simulink model "B_durham_incremental_example"  (R2017a)
settings: Solver=FixedStepAuto  StartTime=0.0  StopTime=10.0  FixedStep=1  RelTol=1e-3
settings Model: Creator=Luca  LastModifiedBy=Luca

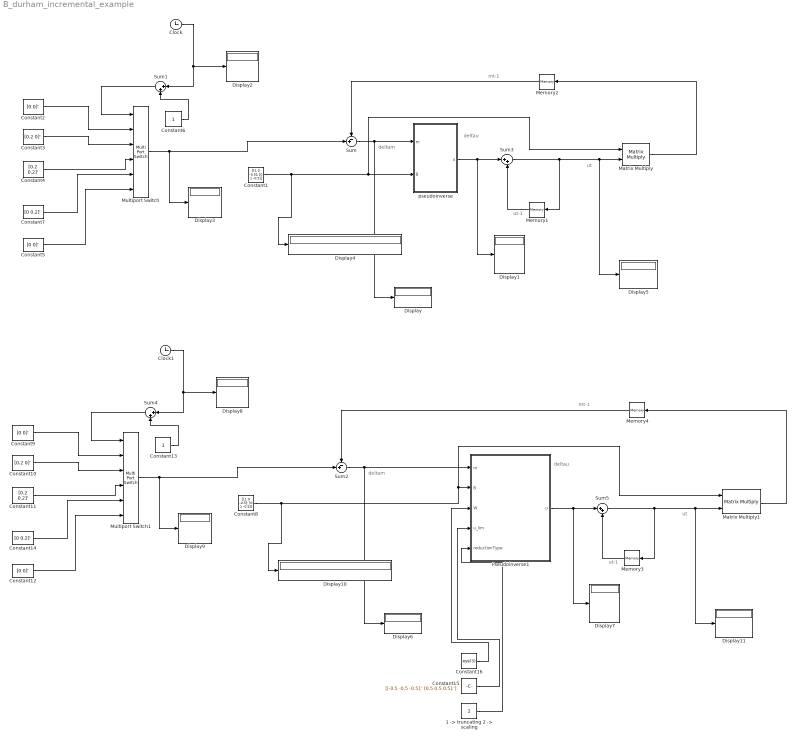
== system B_durham_incremental_example ==
  note: deltam
  note: deltau
  note: ut
  note: ut-1
  note: mt-1
  note: deltam
  note: ut
  note: ut-1
  note: deltau
  note: mt-1
  "1 -> truncating 2 -> scaling" : Constant  Value=2
  Clock : Clock
  Clock1 : Clock
  Constant1 : Constant  Value=[[1 0 -0.5]; [0 1 -0.5]]
  Constant10 : Constant  Value=[0.2 0]'
  Constant11 : Constant  Value=[0.2 0.2]'
  Constant{2,5,9,12} (4 alike) : Constant  Value=[0 0]'
  Constant13 : Constant
  Constant14 : Constant  Value=[0 0.2]'
  Constant15 : Constant  Value=[[-0.5 -0.5 -0.5].' [0.5 0.5 0.5].']
  Constant16 : Constant  Value=eye(3)
  Constant3 : Constant  Value=[0.2 0]'
  Constant4 : Constant  Value=[0.2 0.2]'
  Constant6 : Constant
  Constant7 : Constant  Value=[0 0.2]'
  Constant8 : Constant  Value=[[1 0 -0.5]; [0 1 -0.5]]
  Display{,1..11} (12 alike) : Display
  Matrix Multiply : Product  Multiplication=Matrix(*)
  Matrix Multiply1 : Product  Multiplication=Matrix(*)
  Memory{1..4} (4 alike) : Memory
  Multiport Switch : MultiPortSwitch  Inputs=5
  Multiport Switch1 : MultiPortSwitch  Inputs=5
  Pseudoinverse1 : MATLAB Function  TreatAsAtomicUnit=on
  Sum : Sum  Inputs=-+|
  Sum{1,3..5} (4 alike) : Sum  Inputs=|++
  Sum2 : Sum  Inputs=-+|
  pseudoinverse : MATLAB Function  TreatAsAtomicUnit=on
  wires:
  Memory1/1 -> Sum3/2
  Sum/1 -> Display/1, pseudoinverse/1(m)
  pseudoinverse/1(u) -> Display1/1, Sum3/1
  Memory2/1 -> Sum/1
  Matrix Multiply/1 -> Memory2/1
  Sum3/1 -> Display5/1, Matrix Multiply/2, Memory1/1
  Multiport Switch/1 -> Display3/1, Sum/2
  Constant1/1 -> pseudoinverse/2(B), Matrix Multiply/1, Display4/1
  Constant3/1 -> Multiport Switch/3
  Constant2/1 -> Multiport Switch/2
  Constant4/1 -> Multiport Switch/4
  Clock/1 -> Display2/1, Sum1/1
  Sum1/1 -> Multiport Switch/1
  Constant6/1 -> Sum1/2
  Constant5/1 -> Multiport Switch/6
  Constant7/1 -> Multiport Switch/5
  Matrix Multiply1/1 -> Memory4/1
  Clock1/1 -> Display8/1, Sum4/1
  Constant14/1 -> Multiport Switch1/5
  Constant12/1 -> Multiport Switch1/6
  Sum4/1 -> Multiport Switch1/1
  Memory4/1 -> Sum2/1
  Constant13/1 -> Sum4/2
  Constant9/1 -> Multiport Switch1/2
  Constant10/1 -> Multiport Switch1/3
  Multiport Switch1/1 -> Display9/1, Sum2/2
  Constant8/1 -> Pseudoinverse1/2(B), Matrix Multiply1/1, Display10/1
  Constant11/1 -> Multiport Switch1/4
  Sum5/1 -> Display11/1, Matrix Multiply1/2, Memory3/1
  Memory3/1 -> Sum5/2
  Sum2/1 -> Pseudoinverse1/1(m), Display6/1
  Pseudoinverse1/1(u) -> Display7/1, Sum5/1
  Constant16/1 -> Pseudoinverse1/3(W)
  Constant15/1 -> Pseudoinverse1/4(u_lim)
  "1 -> truncating 2 -> scaling"/1 -> Pseudoinverse1/5(reductionType)

== matlab function B_durham_incremental_example/pseudoinverse ==
  data: m input; u output; B input
function u = Pseudoinverse(m,B)
u = B'*inv(B*B')*m;
end

== matlab function B_durham_incremental_example/Pseudoinverse1 ==
  data: m input; u output; B input; W input; u_lim input; reductionType input
function u = Pseudoinverse(m, B, W, u_lim, reductionType)
coder.varsize('u_index', 'Br', 'Wr', 'u_sat');

%check if the matrices are correct
    if not(isequal(size(u_lim,1),size(B,2),size(W,1),size(W,2))...
       && isequal(length(m),size(B,1)))
        error ('input matrix dimensions do not match')
    end
    
%assign to every equation an index    
    u_index = [1:length(u_lim)].';
    
%check the type of system and then compute the pseudoinverse 1st step
    order = size(B,2)-size(B,1);

    if order > 0 %over-determined, solution that minimizes the 2norm
        u = inv(W)*B'*inv(B*inv(W)*B')*m;
    elseif order < 0 %under-determined, solution that minimizes the error
        u = inv(B'*B)*B'*m;   
    else %order = 0, sqared thus invertiBrle
        u = inv(B)*m;
    end

%deifne u_sat vector
    u_sat = zeros(length(u),1);
    
%check if the first iteration solution is correct then return    
    if not(any(u < u_lim(:,1))||any(u > u_lim(:,2)))  
        return
    end
    
%The software continues only if the solution has to be reduced
%reduce their value
    switch reductionType
        case 1 %truncation
            %takes note of which one are out of their bounds
                u_sat(u < u_lim(:,1)) = 1;
                u_sat(u > u_lim(:,2)) = 1;
                
            %trucate
                u = min(u, u_lim(:,2));
                u = max(u, u_lim(:,1));

        case 2 %scaling solution -> direction preserving
            %reduce
                a = zeros(length(u),1);

                for i = 1:length(u)
                    if u(i)>0
                       a(i) = u(i)/u_lim(i,2);
                    elseif u(i)<0
                       a(i) = u(i)/u_lim(i,1);
                    else
                       a(i) = 0; 
                    end          
                end
                a_max = max(a);
                u = u/a_max;
            
            %takes note of which one are out of their bounds
                u_sat(u == u_lim(:,2)) = 1;
                u_sat(u == u_lim(:,1)) = 1;
            
    end
    
return
    
end
